simulink model "CM4_SPI_Framework"  (R2020b)
settings: Solver=FixedStepDiscrete  StartTime=0.0  StopTime=inf  FixedStep=0.001  RelTol=1e-3  EnableMultiTasking=on
libraries: simulink x9, raspberrypiCommlib x4, embdlinuxlib x1
settings Model: ModifiedByFormat=The MathWorks Inc.  SimulationMode=external  EnablePacing=on  Creator=The MathWorks, Inc.  LastModifiedBy=The MathWorks Inc.
settings SolverCC: PositivePriorityOrder=on
settings DataIOCC: LimitDataPoints=on  SaveFormat=Array  ReturnWorkspaceOutputs=off
settings OptimizationCC: LifeSpan=1  MaxStackSize=64
settings DebuggingCC: UnderspecifiedInitializationDetection=Classic  MergeDetectMultiDrivingBlocksExec=none  SolverPrmCheckMsg=warning  AllowSymbolicDim=off  SFUnexpectedBacktrackingDiag=warning  SFNoUnconditionalDefaultTransitionDiag=warning  SFExecutionAtInitializationDiag=none  ArithmeticOperatorsInVariantConditions=warning
settings HardwareCC: ProdBitPerPointer=32  ProdBitPerSizeT=32  ProdBitPerPtrDiffT=32  ProdLargestAtomicInteger=Long  ProdLargestAtomicFloat=Double  ProdWordSize=32  ProdLongLongMode=on  ProdHWDeviceType=ARM Compatible->ARM Cortex
settings SFSimCC: SimUseLocalCustomCode=off  MATLABDynamicMemAlloc=off  CustomCodeUndefinedFunction=UseInterfaceOnly
settings RTWCC: Description=Embedded Coder  SystemTargetFile=ert.tlc  HardwareBoard=Raspberry Pi  TemplateMakefile=ert_default_tmf  RTWUseLocalCustomCode=off  Toolchain=GNU GCC Raspberry Pi
settings CodeAppCC: StateflowObjectComments=on
settings ERTTargetCC: MultiwordLength=2048  ERTCustomFileBanners=off  MatFileLogging=on  SupportContinuousTime=on  SupportNonInlinedSFcns=on  RemoveResetFunc=off  ModelStepFunctionPrototypeControlCompliant=off  ConvertIfToSwitch=off  SuppressUnreachableDefaultCases=off
settings ConfigComp: CovMetricSettings=dw  CovSaveCumulativeToWorkspaceVar=on  CovSaveSingleToWorkspaceVar=on  CovExternalEMLEnable=off  CovSFcnEnable=off

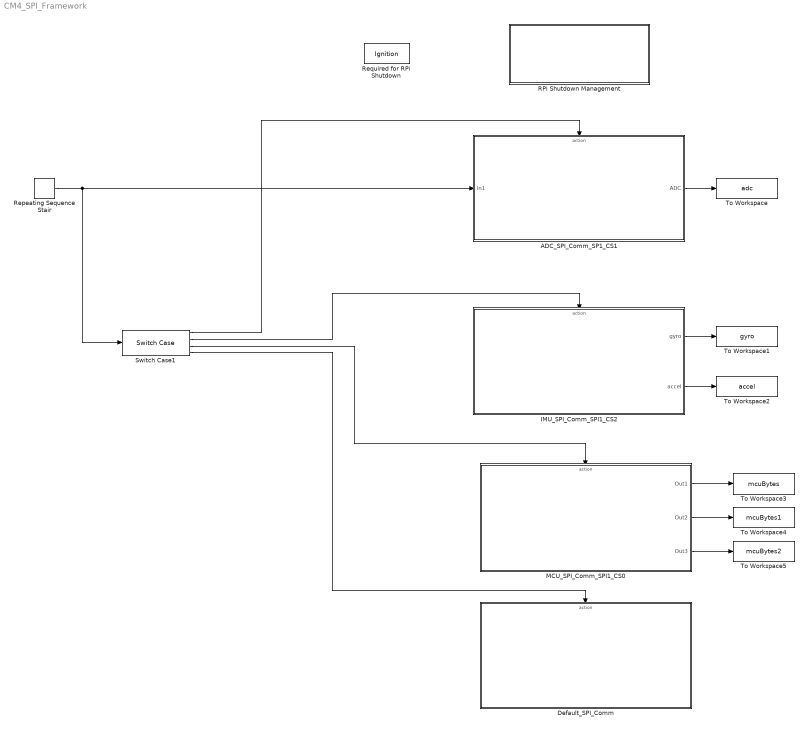
== system CM4_SPI_Framework ==
  ADC_SPI_Comm_SP1_CS1 : Subsystem  TreatAsAtomicUnit=on
  Default_SPI_Comm : Subsystem  TreatAsAtomicUnit=on
  IMU_SPI_Comm_SPI1_CS2 : Subsystem  TreatAsAtomicUnit=on
  MCU_SPI_Comm_SPI1_CS0 : Subsystem  TreatAsAtomicUnit=on
  RPi Shutdown Management : Subsystem
  Repeating Sequence Stair : simulink/Sources/Repeating Sequence Stair  OutValues=(0:12)'  tsamp=-1  OutMin=[]  OutMax=[]  OutDataTypeStr=double  OutputDataTypeScalingMode=double  OutDataType=fixdt(0,8)  ConRadixGroup=Best Precision: Vector-wise  OutScaling=2^-12
  Required for RPi Shutdown : DataStoreMemory  DataStoreName=Ignition  ReadBeforeWriteMsg=warning  WriteAfterWriteMsg=warning  WriteAfterReadMsg=warning  ShowAdditionalParam=off  OutDataTypeStr=uint8
  Switch Case1 : SwitchCase  CaseConditions={[1,2,3,4,5,6],7,8}
  To Workspace : ToWorkspace  VariableName=adc  SampleTime=-1
      settings: Save2DSignal=2-D array (concatenate along first dimension)
  To Workspace1 : ToWorkspace  VariableName=gyro  SampleTime=-1
      settings: Save2DSignal=2-D array (concatenate along first dimension)
  To Workspace2 : ToWorkspace  VariableName=accel  SampleTime=-1
      settings: Save2DSignal=2-D array (concatenate along first dimension)
  To Workspace3 : ToWorkspace  VariableName=mcuBytes  SampleTime=-1
      settings: Save2DSignal=2-D array (concatenate along first dimension)
  To Workspace4 : ToWorkspace  VariableName=mcuBytes1  SampleTime=-1
      settings: Save2DSignal=2-D array (concatenate along first dimension)
  To Workspace5 : ToWorkspace  VariableName=mcuBytes2  SampleTime=-1
      settings: Save2DSignal=2-D array (concatenate along first dimension)
  wires:
  Repeating Sequence Stair/1 -> ADC_SPI_Comm_SP1_CS1/1(In1), Switch Case1/1
  Switch Case1/1 -> ADC_SPI_Comm_SP1_CS1/Action
  Switch Case1/2 -> IMU_SPI_Comm_SPI1_CS2/Action
  Switch Case1/4 -> Default_SPI_Comm/Action
  ADC_SPI_Comm_SP1_CS1/1(ADC) -> To Workspace/1
  IMU_SPI_Comm_SPI1_CS2/2(accel) -> To Workspace2/1
  IMU_SPI_Comm_SPI1_CS2/1(gyro) -> To Workspace1/1
  MCU_SPI_Comm_SPI1_CS0/3(Out3) -> To Workspace5/1
  MCU_SPI_Comm_SPI1_CS0/2(Out2) -> To Workspace4/1
  MCU_SPI_Comm_SPI1_CS0/1(Out1) -> To Workspace3/1
  Switch Case1/3 -> MCU_SPI_Comm_SPI1_CS0/Action

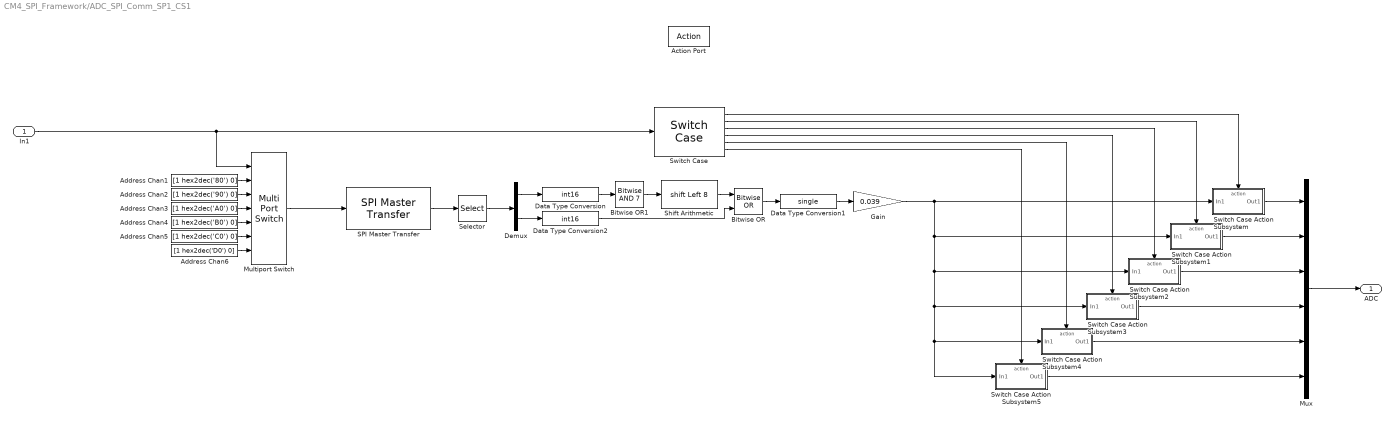
== system CM4_SPI_Framework/ADC_SPI_Comm_SP1_CS1 ==
  In1 : Inport
  Action Port : ActionPort  ActionPortLabel=case [ 1 2 3 4 5 6 ]:
  Address Chan1 : Constant  Value=[1 hex2dec('80') 0]  OutDataTypeStr=uint8
  Address Chan2 : Constant  Value=[1 hex2dec('90') 0]  OutDataTypeStr=uint8
  Address Chan3 : Constant  Value=[1 hex2dec('A0') 0]  OutDataTypeStr=uint8
  Address Chan4 : Constant  Value=[1 hex2dec('B0') 0]  OutDataTypeStr=uint8
  Address Chan5 : Constant  Value=[1 hex2dec('C0') 0]  OutDataTypeStr=uint8
  Address Chan6 : Constant  Value=[1 hex2dec('D0') 0]  OutDataTypeStr=uint8
  Bitwise OR : simulink/Logic and Bit Operations/Bitwise Operator  logicop=OR  UseBitMask=off  NumInputPorts=2  BitMask=bin2dec('11011001')  BitMaskRealWorld=Stored Integer
  Bitwise OR1 : simulink/Logic and Bit Operations/Bitwise Operator  logicop=AND  UseBitMask=on  BitMask=7  BitMaskRealWorld=Stored Integer
  Data Type Conversion : DataTypeConversion  OutDataTypeStr=int16
  Data Type Conversion1 : DataTypeConversion  OutDataTypeStr=single
  Data Type Conversion2 : DataTypeConversion  OutDataTypeStr=int16
  Demux : Demux  Outputs=2
  Gain : Gain  Gain=0.039
  Multiport Switch : MultiPortSwitch  DataPortOrder=Zero-based contiguous  Inputs=6  zeroidx=on  OutDataTypeStr=uint8
  Mux : Mux  Inputs=6
  SPI Master Transfer : raspberrypiCommlib/SPI Master Transfer  BoardProperty=Pi 4 Model B  SPIModule=SPI1  Mode=Master  BusSpeed=1000000  Pin=uint32(0)  FirstBitToTransfer=Most significant bit (MSB)  ClockMode=0  BlockFunction=Transfer  RegisterAddress=0  OutputDataType=int8  OutputDataLength=1  SSPin=CS1
      settings: SourceProductBaseCode=RASPPI
  Selector : Selector  InputPortWidth=3  IndexOptions=Index vector (dialog)  Indices=[2 3]  OutputSizes=1
  Shift Arithmetic : ArithShift  BitShiftNumber=8  BitShiftDirection=Left
  Switch Case : SwitchCase  CaseConditions={0,1,2,3,4,5}  ShowDefaultCase=off
  Switch Case Action Subsystem : Subsystem  TreatAsAtomicUnit=on
  Switch Case Action Subsystem1 : Subsystem  TreatAsAtomicUnit=on
  Switch Case Action Subsystem2 : Subsystem  TreatAsAtomicUnit=on
  Switch Case Action Subsystem3 : Subsystem  TreatAsAtomicUnit=on
  Switch Case Action Subsystem4 : Subsystem  TreatAsAtomicUnit=on
  Switch Case Action Subsystem5 : Subsystem  TreatAsAtomicUnit=on
  ADC : Outport
  wires:
  Switch Case Action Subsystem1/1(Out1) -> Mux/2
  Switch Case/2 -> Switch Case Action Subsystem1/Action
  Address Chan1/1 -> Multiport Switch/2
  Switch Case Action Subsystem3/1(Out1) -> Mux/4
  Bitwise OR/1 -> Data Type Conversion1/1
  Switch Case/5 -> Switch Case Action Subsystem4/Action
  Demux/2 -> Data Type Conversion2/1
  Address Chan3/1 -> Multiport Switch/4
  In1/1 -> Multiport Switch/1, Switch Case/1
  Data Type Conversion1/1 -> Gain/1
  Data Type Conversion/1 -> Bitwise OR1/1
  Switch Case Action Subsystem2/1(Out1) -> Mux/3
  Switch Case Action Subsystem4/1(Out1) -> Mux/5
  Shift Arithmetic/1 -> Bitwise OR/1
  Address Chan6/1 -> Multiport Switch/7
  Multiport Switch/1 -> SPI Master Transfer/1
  Data Type Conversion2/1 -> Bitwise OR/2
  Bitwise OR1/1 -> Shift Arithmetic/1
  Switch Case/1 -> Switch Case Action Subsystem/Action
  SPI Master Transfer/1 -> Selector/1
  Switch Case Action Subsystem/1(Out1) -> Mux/1
  Gain/1 -> Switch Case Action Subsystem5/1(In1), Switch Case Action Subsystem4/1(In1), Switch Case Action Subsystem3/1(In1), Switch Case Action Subsystem2/1(In1), Switch Case Action Subsystem1/1(In1), Switch Case Action Subsystem/1(In1)
  Switch Case/6 -> Switch Case Action Subsystem5/Action
  Demux/1 -> Data Type Conversion/1
  Address Chan4/1 -> Multiport Switch/5
  Selector/1 -> Demux/1
  Address Chan5/1 -> Multiport Switch/6
  Address Chan2/1 -> Multiport Switch/3
  Switch Case/3 -> Switch Case Action Subsystem2/Action
  Switch Case/4 -> Switch Case Action Subsystem3/Action
  Switch Case Action Subsystem5/1(Out1) -> Mux/6
  Mux/1 -> ADC/1

== system CM4_SPI_Framework/Default_SPI_Comm ==
  Action Port : ActionPort  ActionPortLabel=default:
  Subsystem2 : Subsystem
      mask Display:
      | scl=1/4;
      | patch(scl*[0,52,90,54],scl*[16,55,146,146],[16/255,118/255,188/255],'bottom-left');
      | patch(scl*[0,27,82,77,68],scl*[16,0,42,62,69],[46/255,49/255,146/255],'bottom-left');
      | patch(scl*[89,125,90,68],scl*[16,16,146,91],[0,0,0],'bottom-left');
      | disp('Run Once at Startup');

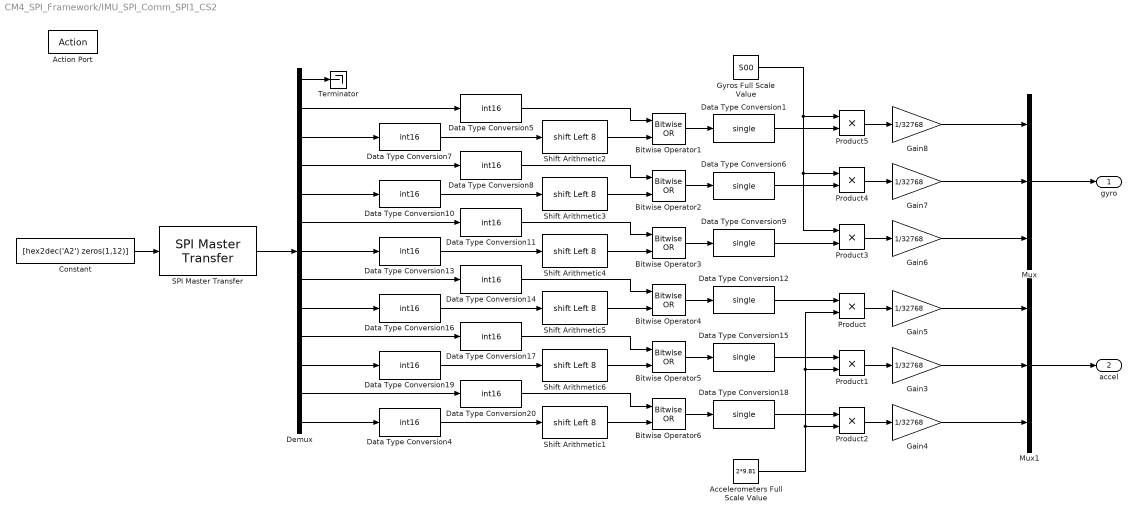
== system CM4_SPI_Framework/IMU_SPI_Comm_SPI1_CS2 ==
  Action Port : ActionPort  ActionPortLabel=case [ 7 ]:
  Accelerometers Full Scale Value : Constant  Value=2*9.81
  Bitwise Operator{1..6} (6 alike) : simulink/Logic and Bit Operations/Bitwise Operator  logicop=OR  UseBitMask=off  NumInputPorts=2  BitMask=bin2dec('11011001')  BitMaskRealWorld=Stored Integer
  Constant : Constant  Value=[hex2dec('A2') zeros(1,12)]  OutDataTypeStr=uint8
  Data Type Conversion{1,6,9,12,15,18} (6 alike) : DataTypeConversion  OutDataTypeStr=single
  Data Type Conversion{4..5,7..8,10..11,13..14,16..17,19..20} (12 alike) : DataTypeConversion  OutDataTypeStr=int16  ConvertRealWorld=Stored Integer (SI)
  Demux : Demux  Outputs=13
  Gain{3..8} (6 alike) : Gain  Gain=1/32768
  Gyros Full Scale Value : Constant  Value=500
  Mux : Mux  Inputs=3
  Mux1 : Mux  Inputs=3
  Product{,1..5} (6 alike) : Product
  SPI Master Transfer : raspberrypiCommlib/SPI Master Transfer  BoardProperty=Pi 4 Model B  SPIModule=SPI1  Mode=Master  BusSpeed=1000000  Pin=uint32(0)  FirstBitToTransfer=Most significant bit (MSB)  ClockMode=0  BlockFunction=Transfer  RegisterAddress=0  OutputDataType=int8  OutputDataLength=1  SSPin=CS2
      settings: SourceProductBaseCode=RASPPI
  Shift Arithmetic{1..6} (6 alike) : ArithShift  BitShiftNumber=8  BitShiftDirection=Left
  Terminator : Terminator
  gyro : Outport
  accel : Outport  Port=2
  wires:
  Demux/5 -> Data Type Conversion10/1
  Product5/1 -> Gain8/1
  Product1/1 -> Gain3/1
  Demux/11 -> Data Type Conversion19/1
  Data Type Conversion8/1 -> Bitwise Operator2/1
  Demux/10 -> Data Type Conversion17/1
  Demux/13 -> Data Type Conversion4/1
  Data Type Conversion16/1 -> Shift Arithmetic5/1
  Shift Arithmetic4/1 -> Bitwise Operator3/2
  Demux/6 -> Data Type Conversion11/1
  Constant/1 -> SPI Master Transfer/1
  Data Type Conversion6/1 -> Product4/2
  Product4/1 -> Gain7/1
  Gain3/1 -> Mux1/2
  Shift Arithmetic3/1 -> Bitwise Operator2/2
  Data Type Conversion4/1 -> Shift Arithmetic1/1
  Product2/1 -> Gain4/1
  Data Type Conversion7/1 -> Shift Arithmetic2/1
  Demux/4 -> Data Type Conversion8/1
  Demux/7 -> Data Type Conversion13/1
  Data Type Conversion10/1 -> Shift Arithmetic3/1
  Data Type Conversion20/1 -> Bitwise Operator6/1
  Demux/9 -> Data Type Conversion16/1
  Demux/12 -> Data Type Conversion20/1
  Data Type Conversion5/1 -> Bitwise Operator1/1
  Data Type Conversion17/1 -> Bitwise Operator5/1
  Shift Arithmetic5/1 -> Bitwise Operator4/2
  Gyros Full Scale Value/1 -> Product5/1, Product4/1, Product3/1
  Shift Arithmetic1/1 -> Bitwise Operator6/2
  Demux/1 -> Terminator/1
  Bitwise Operator5/1 -> Data Type Conversion15/1
  Shift Arithmetic6/1 -> Bitwise Operator5/2
  Data Type Conversion11/1 -> Bitwise Operator3/1
  Data Type Conversion14/1 -> Bitwise Operator4/1
  SPI Master Transfer/1 -> Demux/1
  Bitwise Operator1/1 -> Data Type Conversion1/1
  Data Type Conversion19/1 -> Shift Arithmetic6/1
  Gain4/1 -> Mux1/3
  Bitwise Operator4/1 -> Data Type Conversion12/1
  Demux/3 -> Data Type Conversion7/1
  Data Type Conversion9/1 -> Product3/2
  Shift Arithmetic2/1 -> Bitwise Operator1/2
  Gain8/1 -> Mux/1
  Demux/2 -> Data Type Conversion5/1
  Gain7/1 -> Mux/2
  Data Type Conversion15/1 -> Product1/1
  Bitwise Operator6/1 -> Data Type Conversion18/1
  Data Type Conversion12/1 -> Product/1
  Product/1 -> Gain5/1
  Bitwise Operator3/1 -> Data Type Conversion9/1
  Data Type Conversion13/1 -> Shift Arithmetic4/1
  Data Type Conversion1/1 -> Product5/2
  Accelerometers Full Scale Value/1 -> Product2/2, Product1/2, Product/2
  Gain5/1 -> Mux1/1
  Demux/8 -> Data Type Conversion14/1
  Data Type Conversion18/1 -> Product2/1
  Gain6/1 -> Mux/3
  Product3/1 -> Gain6/1
  Bitwise Operator2/1 -> Data Type Conversion6/1
  Mux/1 -> gyro/1
  Mux1/1 -> accel/1

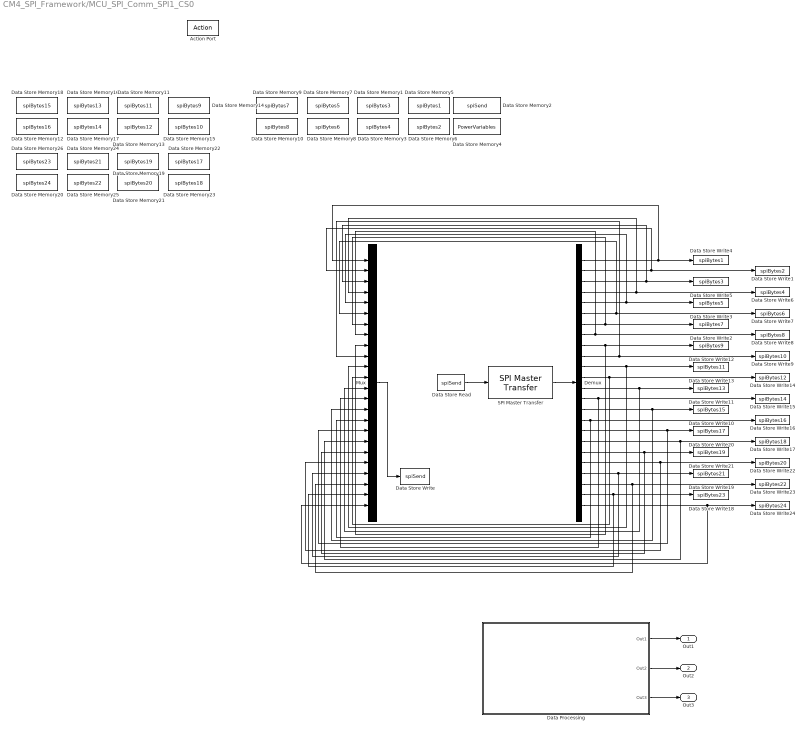
== system CM4_SPI_Framework/MCU_SPI_Comm_SPI1_CS0 ==
  Action Port : ActionPort  ActionPortLabel=case [ 8 ]:
  Data Processing : Subsystem
  Data Store Memory1 : DataStoreMemory  DataStoreName=spiBytes3  ReadBeforeWriteMsg=warning  WriteAfterWriteMsg=warning  WriteAfterReadMsg=warning  InitialValue=[255 255 255 255 255 255 255 255]  ShowAdditionalParam=off  OutDataTypeStr=uint8
  Data Store Memory10 : DataStoreMemory  DataStoreName=spiBytes8  ReadBeforeWriteMsg=warning  WriteAfterWriteMsg=warning  WriteAfterReadMsg=warning  InitialValue=[255 255 255 255 255 255 255 255]  ShowAdditionalParam=off  OutDataTypeStr=uint8
  Data Store Memory11 : DataStoreMemory  DataStoreName=spiBytes11  ReadBeforeWriteMsg=warning  WriteAfterWriteMsg=warning  WriteAfterReadMsg=warning  InitialValue=[255 255 255 255 255 255 255 255]  ShowAdditionalParam=off  OutDataTypeStr=uint8
  Data Store Memory12 : DataStoreMemory  DataStoreName=spiBytes16  ReadBeforeWriteMsg=warning  WriteAfterWriteMsg=warning  WriteAfterReadMsg=warning  InitialValue=[255 255 255 255 255 255 255 255]  ShowAdditionalParam=off  OutDataTypeStr=uint8
  Data Store Memory13 : DataStoreMemory  DataStoreName=spiBytes12  ReadBeforeWriteMsg=warning  WriteAfterWriteMsg=warning  WriteAfterReadMsg=warning  InitialValue=[255 255 255 255 255 255 255 255]  ShowAdditionalParam=off  OutDataTypeStr=uint8
  Data Store Memory14 : DataStoreMemory  DataStoreName=spiBytes9  ReadBeforeWriteMsg=warning  WriteAfterWriteMsg=warning  WriteAfterReadMsg=warning  InitialValue=[255 255 255 255 255 255 255 255]  ShowAdditionalParam=off  OutDataTypeStr=uint8
  Data Store Memory15 : DataStoreMemory  DataStoreName=spiBytes10  ReadBeforeWriteMsg=warning  WriteAfterWriteMsg=warning  WriteAfterReadMsg=warning  InitialValue=[255 255 255 255 255 255 255 255]  ShowAdditionalParam=off  OutDataTypeStr=uint8
  Data Store Memory16 : DataStoreMemory  DataStoreName=spiBytes13  ReadBeforeWriteMsg=warning  WriteAfterWriteMsg=warning  WriteAfterReadMsg=warning  InitialValue=[255 255 255 255 255 255 255 255]  ShowAdditionalParam=off  OutDataTypeStr=uint8
  Data Store Memory17 : DataStoreMemory  DataStoreName=spiBytes14  ReadBeforeWriteMsg=warning  WriteAfterWriteMsg=warning  WriteAfterReadMsg=warning  InitialValue=[255 255 255 255 255 255 255 255]  ShowAdditionalParam=off  OutDataTypeStr=uint8
  Data Store Memory18 : DataStoreMemory  DataStoreName=spiBytes15  ReadBeforeWriteMsg=warning  WriteAfterWriteMsg=warning  WriteAfterReadMsg=warning  InitialValue=[255 255 255 255 255 255 255 255]  ShowAdditionalParam=off  OutDataTypeStr=uint8
  Data Store Memory19 : DataStoreMemory  DataStoreName=spiBytes19  ReadBeforeWriteMsg=warning  WriteAfterWriteMsg=warning  WriteAfterReadMsg=warning  InitialValue=[255 255 255 255 255 255 255 255]  ShowAdditionalParam=off  OutDataTypeStr=uint8
  Data Store Memory2 : DataStoreMemory  DataStoreName=spiSend  ReadBeforeWriteMsg=warning  WriteAfterWriteMsg=warning  WriteAfterReadMsg=warning  InitialValue=zeros(1,192)  ShowAdditionalParam=off  OutDataTypeStr=uint8
  Data Store Memory20 : DataStoreMemory  DataStoreName=spiBytes24  ReadBeforeWriteMsg=warning  WriteAfterWriteMsg=warning  WriteAfterReadMsg=warning  InitialValue=[255 255 255 255 255 255 255 255]  ShowAdditionalParam=off  OutDataTypeStr=uint8
  Data Store Memory21 : DataStoreMemory  DataStoreName=spiBytes20  ReadBeforeWriteMsg=warning  WriteAfterWriteMsg=warning  WriteAfterReadMsg=warning  InitialValue=[255 255 255 255 255 255 255 255]  ShowAdditionalParam=off  OutDataTypeStr=uint8
  Data Store Memory22 : DataStoreMemory  DataStoreName=spiBytes17  ReadBeforeWriteMsg=warning  WriteAfterWriteMsg=warning  WriteAfterReadMsg=warning  InitialValue=[255 255 255 255 255 255 255 255]  ShowAdditionalParam=off  OutDataTypeStr=uint8
  Data Store Memory23 : DataStoreMemory  DataStoreName=spiBytes18  ReadBeforeWriteMsg=warning  WriteAfterWriteMsg=warning  WriteAfterReadMsg=warning  InitialValue=[255 255 255 255 255 255 255 255]  ShowAdditionalParam=off  OutDataTypeStr=uint8
  Data Store Memory24 : DataStoreMemory  DataStoreName=spiBytes21  ReadBeforeWriteMsg=warning  WriteAfterWriteMsg=warning  WriteAfterReadMsg=warning  InitialValue=[255 255 255 255 255 255 255 255]  ShowAdditionalParam=off  OutDataTypeStr=uint8
  Data Store Memory25 : DataStoreMemory  DataStoreName=spiBytes22  ReadBeforeWriteMsg=warning  WriteAfterWriteMsg=warning  WriteAfterReadMsg=warning  InitialValue=[255 255 255 255 255 255 255 255]  ShowAdditionalParam=off  OutDataTypeStr=uint8
  Data Store Memory26 : DataStoreMemory  DataStoreName=spiBytes23  ReadBeforeWriteMsg=warning  WriteAfterWriteMsg=warning  WriteAfterReadMsg=warning  InitialValue=[255 255 255 255 255 255 255 255]  ShowAdditionalParam=off  OutDataTypeStr=uint8
  Data Store Memory3 : DataStoreMemory  DataStoreName=spiBytes4  ReadBeforeWriteMsg=warning  WriteAfterWriteMsg=warning  WriteAfterReadMsg=warning  InitialValue=[255 255 255 255 255 255 255 255]  ShowAdditionalParam=off  OutDataTypeStr=uint8
  Data Store Memory4 : DataStoreMemory  DataStoreName=PowerVariables  ReadBeforeWriteMsg=warning  WriteAfterWriteMsg=warning  WriteAfterReadMsg=warning  InitialValue=[0 0 0 0 0 0 0 0]  ShowAdditionalParam=off  OutDataTypeStr=uint8
  Data Store Memory5 : DataStoreMemory  DataStoreName=spiBytes1  ReadBeforeWriteMsg=warning  WriteAfterWriteMsg=warning  WriteAfterReadMsg=warning  InitialValue=[255 255 255 255 255 255 255 255]  ShowAdditionalParam=off  OutDataTypeStr=uint8
  Data Store Memory6 : DataStoreMemory  DataStoreName=spiBytes2  ReadBeforeWriteMsg=warning  WriteAfterWriteMsg=warning  WriteAfterReadMsg=warning  InitialValue=[255 255 255 255 255 255 255 255]  ShowAdditionalParam=off  OutDataTypeStr=uint8
  Data Store Memory7 : DataStoreMemory  DataStoreName=spiBytes5  ReadBeforeWriteMsg=warning  WriteAfterWriteMsg=warning  WriteAfterReadMsg=warning  InitialValue=[255 255 255 255 255 255 255 255]  ShowAdditionalParam=off  OutDataTypeStr=uint8
  Data Store Memory8 : DataStoreMemory  DataStoreName=spiBytes6  ReadBeforeWriteMsg=warning  WriteAfterWriteMsg=warning  WriteAfterReadMsg=warning  InitialValue=[255 255 255 255 255 255 255 255]  ShowAdditionalParam=off  OutDataTypeStr=uint8
  Data Store Memory9 : DataStoreMemory  DataStoreName=spiBytes7  ReadBeforeWriteMsg=warning  WriteAfterWriteMsg=warning  WriteAfterReadMsg=warning  InitialValue=[255 255 255 255 255 255 255 255]  ShowAdditionalParam=off  OutDataTypeStr=uint8
  Data Store Read : DataStoreRead  DataStoreName=spiSend
  Data Store Write : DataStoreWrite  DataStoreName=spiSend
  Data Store Write1 : DataStoreWrite  DataStoreName=spiBytes2
  Data Store Write10 : DataStoreWrite  DataStoreName=spiBytes15
  Data Store Write11 : DataStoreWrite  DataStoreName=spiBytes13
  Data Store Write12 : DataStoreWrite  DataStoreName=spiBytes9
  Data Store Write13 : DataStoreWrite  DataStoreName=spiBytes11
  Data Store Write14 : DataStoreWrite  DataStoreName=spiBytes12
  Data Store Write15 : DataStoreWrite  DataStoreName=spiBytes14
  Data Store Write16 : DataStoreWrite  DataStoreName=spiBytes16
  Data Store Write17 : DataStoreWrite  DataStoreName=spiBytes18
  Data Store Write18 : DataStoreWrite  DataStoreName=spiBytes23
  Data Store Write19 : DataStoreWrite  DataStoreName=spiBytes21
  Data Store Write2 : DataStoreWrite  DataStoreName=spiBytes7
  Data Store Write20 : DataStoreWrite  DataStoreName=spiBytes17
  Data Store Write21 : DataStoreWrite  DataStoreName=spiBytes19
  Data Store Write22 : DataStoreWrite  DataStoreName=spiBytes20
  Data Store Write23 : DataStoreWrite  DataStoreName=spiBytes22
  Data Store Write24 : DataStoreWrite  DataStoreName=spiBytes24
  Data Store Write3 : DataStoreWrite  DataStoreName=spiBytes5
  Data Store Write4 : DataStoreWrite  DataStoreName=spiBytes1
  Data Store Write5 : DataStoreWrite  DataStoreName=spiBytes3
  Data Store Write6 : DataStoreWrite  DataStoreName=spiBytes4
  Data Store Write7 : DataStoreWrite  DataStoreName=spiBytes6
  Data Store Write8 : DataStoreWrite  DataStoreName=spiBytes8
  Data Store Write9 : DataStoreWrite  DataStoreName=spiBytes10
  Demux : Demux  Outputs=24
  Mux : Mux  Inputs=24
  SPI Master Transfer : raspberrypiCommlib/SPI Master Transfer  BoardProperty=Pi 4 Model B  SPIModule=SPI1  Mode=Master  BusSpeed=1000000  Pin=SPI0_CE0  FirstBitToTransfer=Most significant bit (MSB)  ClockMode=2  BlockFunction=Transfer  RegisterAddress=0  OutputDataType=int8  OutputDataLength=1  SSPin=CS0
      settings: SourceProductBaseCode=RASPPI
  Out1 : Outport
  Out2 : Outport  Port=2
  Out3 : Outport  Port=3
  wires:
  Demux/13 -> Mux/13, Data Store Write11/1
  Demux/24 -> Mux/24, Data Store Write24/1
  Demux/17 -> Mux/17, Data Store Write20/1
  Demux/8 -> Mux/8, Data Store Write8/1
  Demux/19 -> Mux/19, Data Store Write21/1
  Demux/23 -> Mux/23, Data Store Write18/1
  Demux/10 -> Mux/10, Data Store Write9/1
  Demux/20 -> Mux/20, Data Store Write22/1
  Demux/9 -> Mux/9, Data Store Write12/1
  Demux/1 -> Mux/1, Data Store Write4/1
  Demux/12 -> Mux/12, Data Store Write14/1
  Demux/16 -> Mux/16, Data Store Write16/1
  Demux/22 -> Mux/22, Data Store Write23/1
  Demux/11 -> Mux/11, Data Store Write13/1
  Demux/7 -> Mux/7, Data Store Write2/1
  Demux/2 -> Mux/2, Data Store Write1/1
  Data Store Read/1 -> SPI Master Transfer/1
  Demux/4 -> Mux/4, Data Store Write6/1
  Demux/21 -> Mux/21, Data Store Write19/1
  Demux/14 -> Mux/14, Data Store Write15/1
  Demux/6 -> Mux/6, Data Store Write7/1
  Demux/15 -> Mux/15, Data Store Write10/1
  Demux/3 -> Mux/3, Data Store Write5/1
  Mux/1 -> Data Store Write/1
  Demux/18 -> Mux/18, Data Store Write17/1
  Demux/5 -> Mux/5, Data Store Write3/1
  SPI Master Transfer/1 -> Demux/1
  Data Processing/1(Out1) -> Out1/1
  Data Processing/2(Out2) -> Out2/1
  Data Processing/3(Out3) -> Out3/1

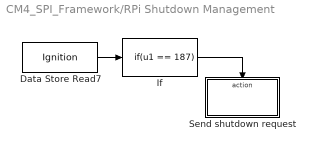
== system CM4_SPI_Framework/RPi Shutdown Management ==
  Data Store Read7 : DataStoreRead  DataStoreName=Ignition
  If : If  IfExpression=u1 == 187  ShowElse=off
  Send shutdown request : Subsystem  TreatAsAtomicUnit=on
  wires:
  If/1 -> Send shutdown request/Action
  Data Store Read7/1 -> If/1

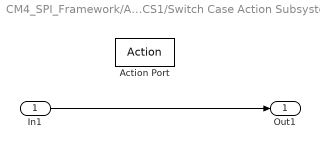
== system CM4_SPI_Framework/ADC_SPI_Comm_SP1_CS1/Switch Case Action Subsystem ==
  In1 : Inport
  Action Port : ActionPort  ActionPortLabel=case [ 0 ]:
  Out1 : Outport
  wires:
  In1/1 -> Out1/1

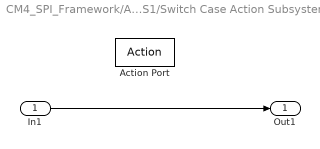
== system CM4_SPI_Framework/ADC_SPI_Comm_SP1_CS1/Switch Case Action Subsystem1 ==
  In1 : Inport
  Action Port : ActionPort  ActionPortLabel=case [ 1 ]:
  Out1 : Outport
  wires:
  In1/1 -> Out1/1

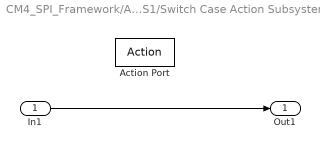
== system CM4_SPI_Framework/ADC_SPI_Comm_SP1_CS1/Switch Case Action Subsystem2 ==
  In1 : Inport
  Action Port : ActionPort  ActionPortLabel=case [ 2 ]:
  Out1 : Outport
  wires:
  In1/1 -> Out1/1

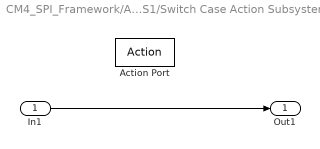
== system CM4_SPI_Framework/ADC_SPI_Comm_SP1_CS1/Switch Case Action Subsystem3 ==
  In1 : Inport
  Action Port : ActionPort  ActionPortLabel=case [ 3 ]:
  Out1 : Outport
  wires:
  In1/1 -> Out1/1

== system CM4_SPI_Framework/ADC_SPI_Comm_SP1_CS1/Switch Case Action Subsystem4 ==
  In1 : Inport
  Action Port : ActionPort  ActionPortLabel=case [ 4 ]:
  Out1 : Outport
  wires:
  In1/1 -> Out1/1

== system CM4_SPI_Framework/ADC_SPI_Comm_SP1_CS1/Switch Case Action Subsystem5 ==
  In1 : Inport
  Action Port : ActionPort  ActionPortLabel=case [ 5 ]:
  Out1 : Outport
  wires:
  In1/1 -> Out1/1

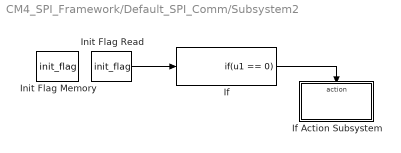
== system CM4_SPI_Framework/Default_SPI_Comm/Subsystem2 ==
  If : If  IfExpression=u1 == 0  ShowElse=off
  If Action Subsystem : Subsystem  TreatAsAtomicUnit=on
  Init Flag Memory : DataStoreMemory  DataStoreName=init_flag  ReadBeforeWriteMsg=warning  WriteAfterWriteMsg=warning  WriteAfterReadMsg=warning  ShowAdditionalParam=off  OutDataTypeStr=uint32
  Init Flag Read : DataStoreRead  DataStoreName=init_flag
  wires:
  Init Flag Read/1 -> If/1
  If/1 -> If Action Subsystem/Action

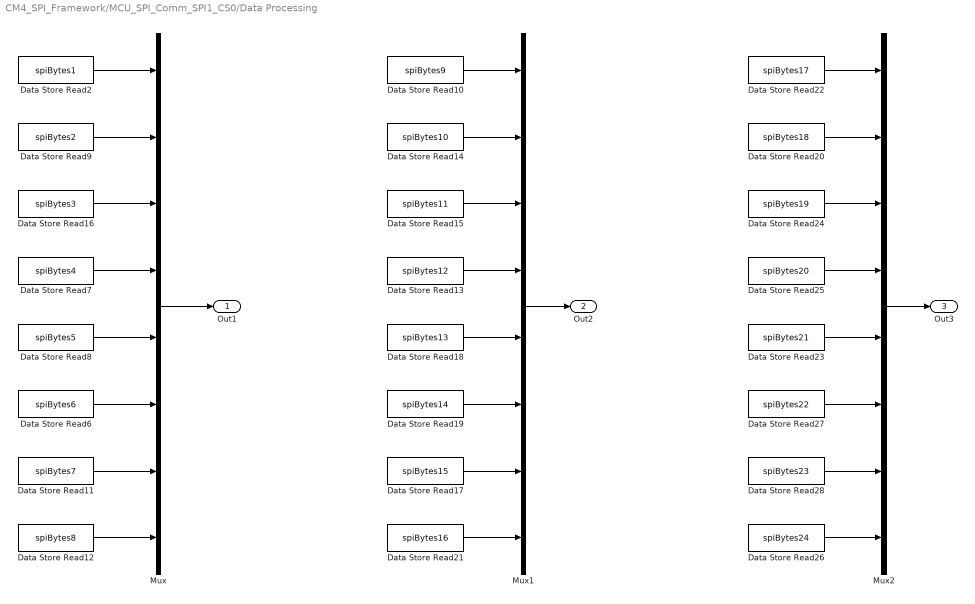
== system CM4_SPI_Framework/MCU_SPI_Comm_SPI1_CS0/Data Processing ==
  Data Store Read10 : DataStoreRead  DataStoreName=spiBytes9
  Data Store Read11 : DataStoreRead  DataStoreName=spiBytes7
  Data Store Read12 : DataStoreRead  DataStoreName=spiBytes8
  Data Store Read13 : DataStoreRead  DataStoreName=spiBytes12
  Data Store Read14 : DataStoreRead  DataStoreName=spiBytes10
  Data Store Read15 : DataStoreRead  DataStoreName=spiBytes11
  Data Store Read16 : DataStoreRead  DataStoreName=spiBytes3
  Data Store Read17 : DataStoreRead  DataStoreName=spiBytes15
  Data Store Read18 : DataStoreRead  DataStoreName=spiBytes13
  Data Store Read19 : DataStoreRead  DataStoreName=spiBytes14
  Data Store Read2 : DataStoreRead  DataStoreName=spiBytes1
  Data Store Read20 : DataStoreRead  DataStoreName=spiBytes18
  Data Store Read21 : DataStoreRead  DataStoreName=spiBytes16
  Data Store Read22 : DataStoreRead  DataStoreName=spiBytes17
  Data Store Read23 : DataStoreRead  DataStoreName=spiBytes21
  Data Store Read24 : DataStoreRead  DataStoreName=spiBytes19
  Data Store Read25 : DataStoreRead  DataStoreName=spiBytes20
  Data Store Read26 : DataStoreRead  DataStoreName=spiBytes24
  Data Store Read27 : DataStoreRead  DataStoreName=spiBytes22
  Data Store Read28 : DataStoreRead  DataStoreName=spiBytes23
  Data Store Read6 : DataStoreRead  DataStoreName=spiBytes6
  Data Store Read7 : DataStoreRead  DataStoreName=spiBytes4
  Data Store Read8 : DataStoreRead  DataStoreName=spiBytes5
  Data Store Read9 : DataStoreRead  DataStoreName=spiBytes2
  Mux : Mux  Inputs=8
  Mux1 : Mux  Inputs=8
  Mux2 : Mux  Inputs=8
  Out1 : Outport
  Out2 : Outport  Port=2
  Out3 : Outport  Port=3
  wires:
  Data Store Read2/1 -> Mux/1
  Data Store Read9/1 -> Mux/2
  Data Store Read16/1 -> Mux/3
  Data Store Read6/1 -> Mux/6
  Data Store Read7/1 -> Mux/4
  Data Store Read8/1 -> Mux/5
  Data Store Read10/1 -> Mux1/1
  Data Store Read11/1 -> Mux/7
  Data Store Read12/1 -> Mux/8
  Data Store Read13/1 -> Mux1/4
  Data Store Read14/1 -> Mux1/2
  Data Store Read15/1 -> Mux1/3
  Data Store Read17/1 -> Mux1/7
  Data Store Read18/1 -> Mux1/5
  Data Store Read19/1 -> Mux1/6
  Data Store Read20/1 -> Mux2/2
  Data Store Read21/1 -> Mux1/8
  Data Store Read22/1 -> Mux2/1
  Data Store Read26/1 -> Mux2/8
  Data Store Read27/1 -> Mux2/6
  Data Store Read28/1 -> Mux2/7
  Data Store Read23/1 -> Mux2/5
  Data Store Read25/1 -> Mux2/4
  Data Store Read24/1 -> Mux2/3
  Mux/1 -> Out1/1
  Mux1/1 -> Out2/1
  Mux2/1 -> Out3/1

== system CM4_SPI_Framework/RPi Shutdown Management/Send shutdown request ==
  Action Port : ActionPort  ActionPortLabel=if(u1 == 187)
  Constant : Constant  Value=187  OutDataTypeStr=uint8
  UDP Send : embdlinuxlib/UDP Send  remoteURL='127.0.0.1'  remotePort=5005  localURL='255.255.255.255'  localPortSource=Automatically determine  localPort=-1  sampletime=-1  blockPlatform=Raspberry Pi  separateLengthPort=0
      settings: SourceProductBaseCode=SC_BEAGLEBONE_BLUE,NVIDIA,RASPPI
  wires:
  Constant/1 -> UDP Send/1

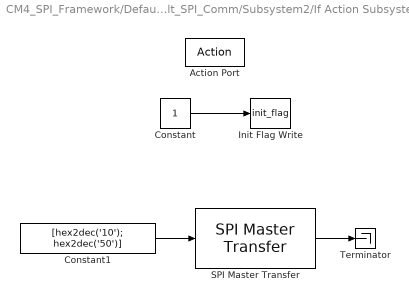
== system CM4_SPI_Framework/Default_SPI_Comm/Subsystem2/If Action Subsystem ==
  Action Port : ActionPort  ActionPortLabel=if(u1 == 0)
  Constant : Constant  OutDataTypeStr=uint32
  Constant1 : Constant  Value=[hex2dec('10'); hex2dec('50')]  OutDataTypeStr=uint8
  Init Flag Write : DataStoreWrite  DataStoreName=init_flag
  SPI Master Transfer : raspberrypiCommlib/SPI Master Transfer  BoardProperty=Pi 4 Model B  SPIModule=SPI1  Mode=Master  BusSpeed=1000000  Pin=uint32(0)  FirstBitToTransfer=Most significant bit (MSB)  ClockMode=0  BlockFunction=Transfer  RegisterAddress=0  OutputDataType=int8  OutputDataLength=1  SSPin=CS2
      settings: SourceProductBaseCode=RASPPI
  Terminator : Terminator
  wires:
  Constant/1 -> Init Flag Write/1
  Constant1/1 -> SPI Master Transfer/1
  SPI Master Transfer/1 -> Terminator/1
